simulink model "modelo_LB"  (R2023b)
settings: Solver=FixedStepDiscrete  StartTime=0  StopTime=50  FixedStep=1  RelTol=1e-3
undefined symbols (not defined in the file): aB, aL, B0, dB, dL, L0
settings Model: Creator=alfre  LastModifiedBy=alfre

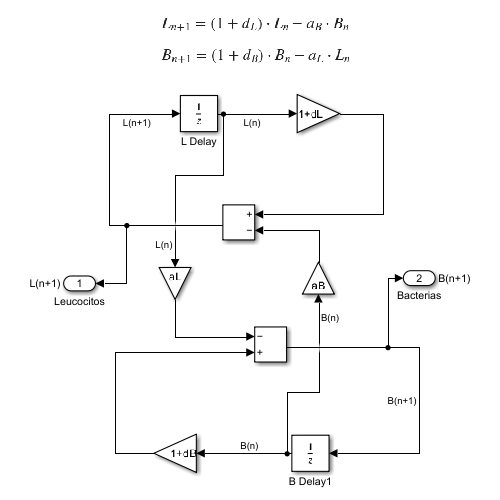
[thumbnail: Simulink's stored preview of the top-level diagram]
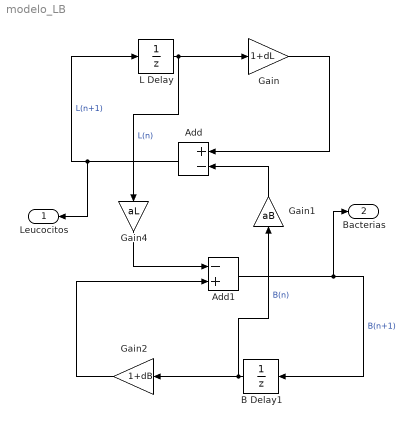
== system modelo_LB ==
  Add : Sum  Inputs=+-
  Add1 : Sum  Inputs=-+
  B Delay1 : UnitDelay  InitialCondition=B0  SampleTime=-1  HasFrameUpgradeWarning=on
  Gain : Gain  Gain=1+dL
  Gain1 : Gain  Gain=aB
  Gain2 : Gain  Gain=1+dB
  Gain4 : Gain  Gain=aL
  L Delay : UnitDelay  InitialCondition=L0  SampleTime=-1  HasFrameUpgradeWarning=on
  Leucocitos : Outport  SignalName=L(n+1)
  Bacterias : Outport  Port=2  SignalName=B(n+1)
  wires:
  Add/1 -> L Delay/1, Leucocitos/1  "L(n+1)"
  L Delay/1 -> Gain4/1, Gain/1  "L(n)"
  Gain/1 -> Add/1
  Add1/1 -> Bacterias/1, B Delay1/1  "B(n+1)"
  B Delay1/1 -> Gain1/1, Gain2/1  "B(n)"
  Gain1/1 -> Add/2
  Gain4/1 -> Add1/1
  Gain2/1 -> Add1/2
